simulink model "movimiento"  (Simulink 7.7)
settings: Solver=ode45  StartTime=0.0  StopTime=10.0  RelTol=1e-3
undefined symbols (not defined in the file or in its folder): jet, none, videoinput
libraries: imaqlib x1, vipsnks x1
settings Model: Creator=bLacko  LastModifiedBy=bLacko

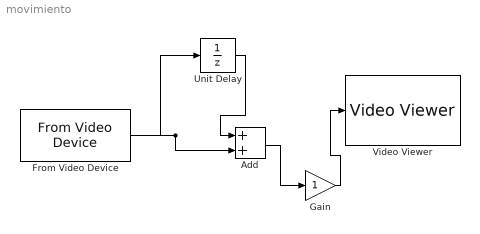
== system movimiento ==
  Add : Sum
  From Video Device : imaqlib/From Video Device  DeviceMenu=winvideo 1 (CyberLink Webcam Splitter)  Device=winvideo 1 (CyberLink Webcam Splitter)  ObjConstructor=videoinput('winvideo', 1)  VideoFormatMenu=RGB24_800x600  VideoFormat=RGB24_320x240  VideoSource=input1  ROIPosition=[0 0 240 320]  EnableHWTrigger=off  TriggerConfiguration=none/none  SampleTime=1/30  OutputPortsMode=One multidimensional signal  DataType=single  CanDoHWTrigger=no  ReturnedColorSpace=rgb  BlockHandle=1926.0001  ROIWidth=320  ROIHeight=240  ROIColumn=0  ROIRow=0  EngXMLPath=C:\Matlab\toolbox\imaq\imaq\private  DevXMLPath=C:\Matlab\toolbox\imaq\imaqadaptors\win64  EngLibPath=C:\Matlab\toolbox\imaq\imaqblks\imaqmex\win64
  Gain : Gain
  Unit Delay : UnitDelay  SampleTime=-1
  Video Viewer : vipsnks/Video Viewer  inputType=Obsolete7b  imagePorts=One multidimensional signal  useColorMap=off  colormapValue=jet(256)  specRange=off  minInputVal=0  maxInputVal=255  FigPos=[219 520 410 300]  AxisZoom=on  trueSizedOnce=off  OpenAtMdlStart=on
  wires:
  From Video Device/1 -> Add/2, Unit Delay/1
  Unit Delay/1 -> Add/1
  Add/1 -> Gain/1
  Gain/1 -> Video Viewer/1
